simulink model "lecture_2_1b"  (R2021a)
settings: Solver=VariableStepAuto  StartTime=0.0  StopTime=10.0  RelTol=1e-3
settings Model: Creator=Admin  LastModifiedBy=Admin

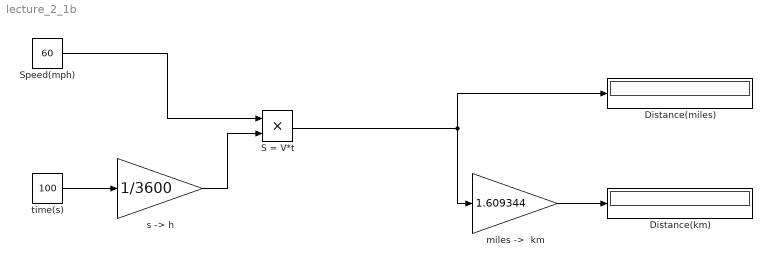
== system lecture_2_1b ==
  "Distance(km) " : Display
  Distance(miles) : Display
  S = V*t : Product
  Speed(mph) : Constant  Value=60
  "miles ->  km  " : Gain  Gain=1.609344
  "s -> h   " : Gain  Gain=1/3600
  time(s) : Constant  Value=100
  wires:
  "miles ->  km  "/1 -> "Distance(km) "/1
  time(s)/1 -> "s -> h   "/1
  "s -> h   "/1 -> S = V*t/2
  Speed(mph)/1 -> S = V*t/1
  S = V*t/1 -> "miles ->  km  "/1, Distance(miles)/1
